simulink model "Integration_Drag_harness"  (R2020b)
settings: Solver=ode4  StartTime=0.0  StopTime=par.sym.Ttot  FixedStep=par.sym.max_dt  MaxStep=par.sym.max_dt  RelTol=1e-3
settings Model: Creator=carar  LastModifiedBy=carar
settings SolverCC: AlgebraicLoopSolver=LineSearch
settings DataIOCC: SaveOutput=off  SaveTime=off  ReturnWorkspaceOutputs=off  TimeSaveName=TIME
settings OptimizationCC: LifeSpan=inf
settings DebuggingCC: UnconnectedInputMsg=none  UnconnectedOutputMsg=none  ArithmeticOperatorsInVariantConditions=warning
settings SFSimCC: CustomCodeUndefinedFunction=UseInterfaceOnly
settings CodeAppCC: GenerateComments=off
settings SimscapeCC: SimscapeNormalizeSystem=off

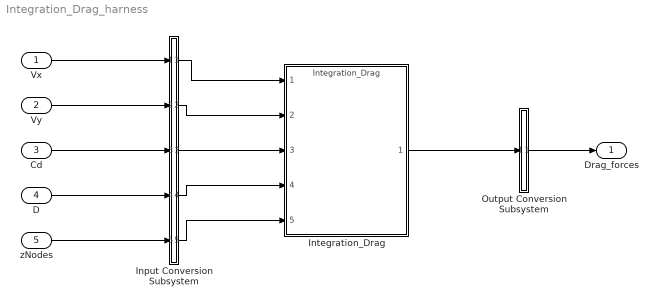
== system Integration_Drag_harness ==
  Vx : Inport  OutDataTypeStr=double  PortDimensions=[10]  SampleTime=0
  Vy : Inport  Port=2  OutDataTypeStr=double  PortDimensions=[10]  SampleTime=0
  Cd : Inport  Port=3  OutDataTypeStr=double  PortDimensions=[1]  SampleTime=0
  D : Inport  Port=4  OutDataTypeStr=double  PortDimensions=[10]  SampleTime=0
  zNodes : Inport  Port=5  OutDataTypeStr=double  PortDimensions=[10]  SampleTime=0
  Input Conversion Subsystem : Subsystem  Tag=__SLT_ICS__  Description=|
      | Signal spec.
      | and routing
      settings: AttributesFormatString=%<Description>
  Integration_Drag : ModelReference  ModelNameDialog=Integration_Drag.slxp  ModelReferenceVersion=5.19  CopyOfModelProtected=on
  Output Conversion Subsystem : Subsystem  Tag=__SLT_OCS__  Description=|
      | Signal spec.
      | and routing
      settings: AttributesFormatString=%<Description>
  Drag_forces : Outport
  wires:
  Vx/1 -> Input Conversion Subsystem/1(Inport_1)
  Vy/1 -> Input Conversion Subsystem/2(Inport_2)
  Cd/1 -> Input Conversion Subsystem/3(Inport_3)
  D/1 -> Input Conversion Subsystem/4(Inport_4)
  zNodes/1 -> Input Conversion Subsystem/5(Inport_5)
  Output Conversion Subsystem/1(Outport_1) -> Drag_forces/1
  Input Conversion Subsystem/1(Outport_1) -> Integration_Drag/1
  Input Conversion Subsystem/2(Outport_2) -> Integration_Drag/2
  Input Conversion Subsystem/3(Outport_3) -> Integration_Drag/3
  Input Conversion Subsystem/4(Outport_4) -> Integration_Drag/4
  Input Conversion Subsystem/5(Outport_5) -> Integration_Drag/5
  Integration_Drag/1 -> Output Conversion Subsystem/1(Inport_1)

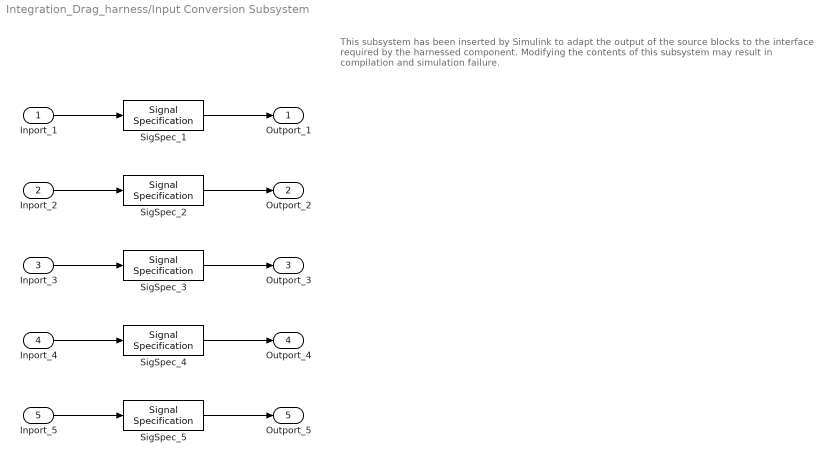
== system Integration_Drag_harness/Input Conversion Subsystem ==
  note: This subsystem has been inserted by Simulink to adapt the output of the source blocks to the interface required by the harnessed component.
      |  Modifying the contents of this subsystem may result in compilation and simulation failure.
  Inport_1 : Inport
  Inport_2 : Inport  Port=2
  Inport_3 : Inport  Port=3
  Inport_4 : Inport  Port=4
  Inport_5 : Inport  Port=5
  SigSpec_{1..2,4..5} (4 alike) : SignalSpecification  OutDataTypeStr=double  Dimensions=[10]  SampleTime=[0, 0]
  SigSpec_3 : SignalSpecification  OutDataTypeStr=double  Dimensions=[1]  SampleTime=[0, 0]
  Outport_1 : Outport
  Outport_2 : Outport  Port=2
  Outport_3 : Outport  Port=3
  Outport_4 : Outport  Port=4
  Outport_5 : Outport  Port=5
  wires:
  SigSpec_1/1 -> Outport_1/1
  Inport_1/1 -> SigSpec_1/1
  SigSpec_2/1 -> Outport_2/1
  Inport_2/1 -> SigSpec_2/1
  SigSpec_3/1 -> Outport_3/1
  Inport_3/1 -> SigSpec_3/1
  SigSpec_4/1 -> Outport_4/1
  Inport_4/1 -> SigSpec_4/1
  SigSpec_5/1 -> Outport_5/1
  Inport_5/1 -> SigSpec_5/1

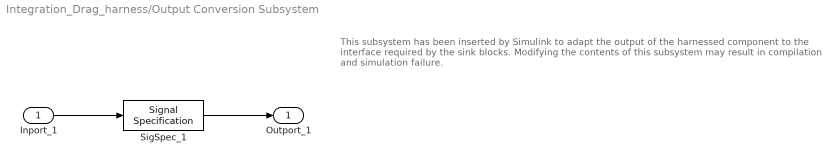
== system Integration_Drag_harness/Output Conversion Subsystem ==
  note: This subsystem has been inserted by Simulink to adapt the output of the harnessed component to the interface required by the sink blocks.
      |  Modifying the contents of this subsystem may result in compilation and simulation failure.
  Inport_1 : Inport
  SigSpec_1 : SignalSpecification  OutDataTypeStr=double  Dimensions=[6]
  Outport_1 : Outport
  wires:
  Inport_1/1 -> SigSpec_1/1
  SigSpec_1/1 -> Outport_1/1
